simulink model "Part_2b"  (R2024a)
settings: Solver=VariableStepAuto  StartTime=0.0  StopTime=20000  RelTol=1e-3
libraries: dspfdesign x1
settings Model: Creator=hemna  LastModifiedBy=sujay

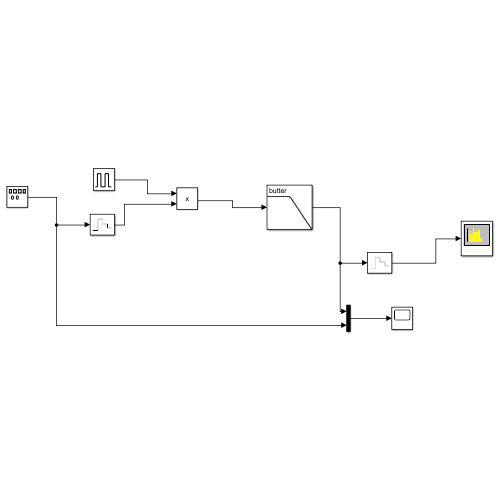
[thumbnail: Simulink's stored preview of the top-level diagram]
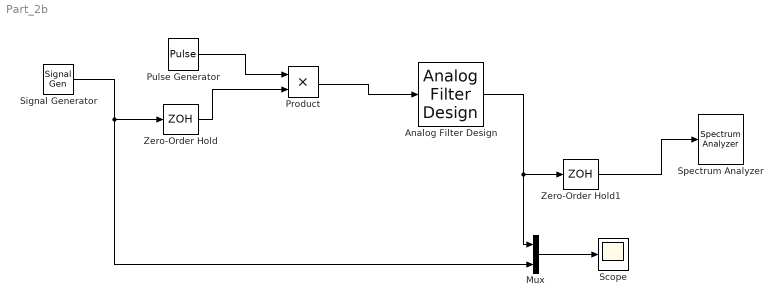
== system Part_2b ==
  Analog Filter Design : dspfdesign/Analog Filter Design  method=Butterworth  filttype=Lowpass  N=10  Wlo=5  Whi=80  Rp=2  Rs=40
  Mux : Mux  Inputs=2
  Product : Product
  Pulse Generator : DiscretePulseGenerator  PulseType=Time based  Period=1  PulseWidth=30
  Scope : Scope
  Signal Generator : SignalGenerator  Frequency=0.8  Units=rad/sec
  Spectrum Analyzer : SpectrumAnalyzer  WindowPosition=[13.000000,42.000000,1536.000000,792.000000,]  ScopeFrameLocation=window  Span=20  StartFrequency=-10  StopFrequency=10  YLimits=[-261.22246287822486,69.20413986881593]  SelectedToolstripTab=spectrumAnalyzerToolstrip.channelMeasurementsTab
  Zero-Order Hold : ZeroOrderHold
  Zero-Order Hold1 : ZeroOrderHold  SampleTime=0.05
  wires:
  Signal Generator/1 -> Mux/2, Zero-Order Hold/1
  Zero-Order Hold/1 -> Product/2
  Pulse Generator/1 -> Product/1
  Mux/1 -> Scope/1
  Zero-Order Hold1/1 -> Spectrum Analyzer/1
  Product/1 -> Analog Filter Design/1
  Analog Filter Design/1 -> Mux/1, Zero-Order Hold1/1
